simulink model "afm_z_dist_sin"  (R2018a)
settings: Solver=VariableStepAuto  StartTime=0.0  StopTime=trun  RelTol=1e-3
libraries: cstblocks x3
settings Model: Creator=arnold  LastModifiedBy=arnold

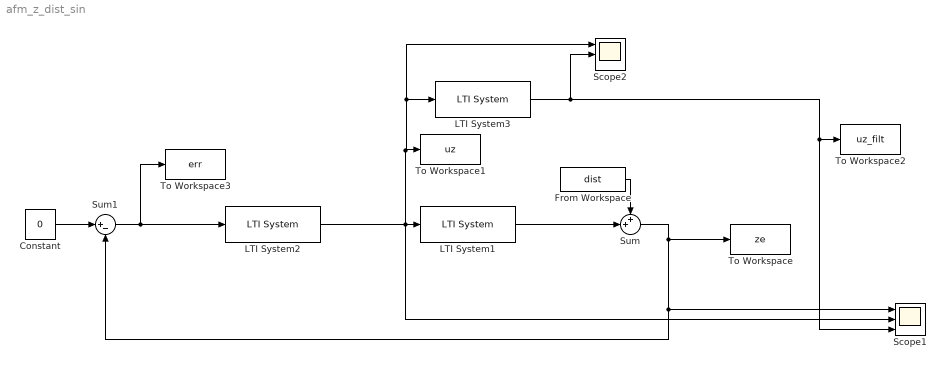
== system afm_z_dist_sin ==
  Constant : Constant  Value=0
  From Workspace : FromWorkspace  VariableName=dist  SampleTime=0
  LTI System1 : cstblocks/LTI System  sys=G  IC=[]
  LTI System2 : cstblocks/LTI System  sys=Dz  IC=[]
  LTI System3 : cstblocks/LTI System  sys=g_filtz  IC=[]
  Scope1 : Scope  NumInputPorts=3
  Scope2 : Scope  NumInputPorts=3
  Sum : Sum  Inputs=++|
  Sum1 : Sum  Inputs=|+-
  To Workspace : ToWorkspace  VariableName=ze  SaveFormat=Timeseries  SampleTime=-1
  To Workspace1 : ToWorkspace  VariableName=uz  SaveFormat=Timeseries  SampleTime=-1
  To Workspace2 : ToWorkspace  VariableName=uz_filt  SaveFormat=Timeseries  SampleTime=-1
  To Workspace3 : ToWorkspace  VariableName=err  SaveFormat=Timeseries  SampleTime=-1
  wires:
  From Workspace/1 -> Sum/1
  LTI System1/1 -> Sum/2
  Constant/1 -> Sum1/1
  Sum1/1 -> LTI System2/1, To Workspace3/1
  LTI System2/1 -> Scope1/2, LTI System3/1, Scope2/1, To Workspace1/1, LTI System1/1
  Sum/1 -> To Workspace/1, Scope1/1, Sum1/2
  LTI System3/1 -> Scope2/2, Scope1/3, To Workspace2/1
